simulink model "StraightWithLeadingCar_cs"  (R2016a)
settings: Solver=ode5  SolverMode=SingleTasking  StartTime=0.0  StopTime=40  FixedStep=1/1000  RelTol=1e-3
PreLoadFcn:
  | mbxruntime.callbacks.PreLoadFcn(bdroot);
PostLoadFcn:
  | mbxruntime.callbacks.PostLoadFcn(bdroot);
InitFcn:
  | mbxruntime.callbacks.InitFcn(bdroot);
StartFcn:
  | mbxruntime.callbacks.StartFcn(bdroot);
StopFcn:
  | mbxruntime.callbacks.StopFcn(bdroot);
model workspace (MAT data in the model file):
  mbox_table : struct (value not decoded)
  model_closed = 0
  sim_status = 0
values from neighbouring files (symbols this model uses):
  ACCDuration = 5    [PreScan_Runscript.m]
  V0 = ACCArray(2*ACCCasei-1)    [PreScan_Runscript.m]
  V1 = ACCArray(2*ACCCasei)    [PreScan_Runscript.m]
  VAccuracyIn = 0.8    [PreScan_Runscript.m]
  VDurationIn = 2    [PreScan_Runscript.m]
  VPIDIn = ACCArray(2*ACCCasei-1)    [PreScan_Runscript.m]
  VToleranceIn = 1    [PreScan_Runscript.m]
undefined symbols (not defined in the file or in its folder): ADASID, BMotor1, BMotor2, BrkDelayTime, DControlB, Delay1, Delay2, DiscIntNeverNeededParam, IControlB, JMotor1, JMotor2, mbxruntime, PControlB, PreScanCarSimLoadFcn, ratioGearF, ratioGearR, tabledata, TorqDelayTime, Tstep
undefined symbols (not defined in the file): SteeringColumn, SteeringWheel, WheelL0, WheelL1, WheelR0, WheelR1
libraries: simulink x14, simulink_extras x11, PreScanSimulinkLibrary x9, MyLib x3, Solver_SF x2, PreScanUsefulBlocks x2, pil_lib x1
(part 12 of 12)

== system StraightWithLeadingCar_cs/Roewe_550_S_Sedan_1/CarSim_Vehicle/CarSim2PreScan_BUS/Wheel/Convert CarSim to PreScan Wheel Position/Transformation_WheelGlobal2WheelLocal/PreScan_WheelShiftFR/pos_ini_Visu ==
  Constant : Constant  Value=x_ini_VRML
  Constant1 : Constant  Value=y_ini_VRML
  Constant2 : Constant  Value=TyreRadius-cogZOffset
  Mux1 : Mux  Inputs=3
  pos_ini_Visu : Outport
  wires:
  Constant/1 -> Mux1/1
  Mux1/1 -> pos_ini_Visu/1
  Constant1/1 -> Mux1/2
  Constant2/1 -> Mux1/3

== system StraightWithLeadingCar_cs/Roewe_550_S_Sedan_1/CarSim_Vehicle/CarSim2PreScan_BUS/Wheel/Convert CarSim to PreScan Wheel Position/Transformation_WheelGlobal2WheelLocal/PreScan_WheelShiftRL/pos_ini_Visu ==
  Constant : Constant  Value=-x_ini_VRML
  Constant1 : Constant  Value=y_ini_VRML
  Constant2 : Constant  Value=TyreRadius-cogZOffset
  Mux1 : Mux  Inputs=3
  pos_ini_Visu : Outport
  wires:
  Constant/1 -> Mux1/1
  Mux1/1 -> pos_ini_Visu/1
  Constant1/1 -> Mux1/2
  Constant2/1 -> Mux1/3

== system StraightWithLeadingCar_cs/Roewe_550_S_Sedan_1/CarSim_Vehicle/CarSim2PreScan_BUS/Wheel/Convert CarSim to PreScan Wheel Position/Transformation_WheelGlobal2WheelLocal/PreScan_WheelShiftRR/pos_ini_Visu ==
  Constant : Constant  Value=-x_ini_VRML
  Constant1 : Constant  Value=y_ini_VRML
  Constant2 : Constant  Value=TyreRadius-cogZOffset
  Mux1 : Mux  Inputs=3
  pos_ini_Visu : Outport
  wires:
  Constant/1 -> Mux1/1
  Mux1/1 -> pos_ini_Visu/1
  Constant1/1 -> Mux1/2
  Constant2/1 -> Mux1/3

== system StraightWithLeadingCar_cs/Roewe_550_S_Sedan_1/Subsystem1/CarSim2PreScan_BUS/Wheel/Convert CarSim to PreScan Wheel Position/Transformation_WheelGlobal2WheelLocal/PreScan_WheelShiftFL/pos_ini_Visu ==
  Constant : Constant  Value=x_ini_VRML
  Constant1 : Constant  Value=y_ini_VRML
  Constant2 : Constant  Value=TyreRadius-cogZOffset
  Mux1 : Mux  Inputs=3
  pos_ini_Visu : Outport
  wires:
  Constant2/1 -> Mux1/3
  Constant1/1 -> Mux1/2
  Mux1/1 -> pos_ini_Visu/1
  Constant/1 -> Mux1/1

== system StraightWithLeadingCar_cs/Roewe_550_S_Sedan_1/Subsystem1/CarSim2PreScan_BUS/Wheel/Convert CarSim to PreScan Wheel Position/Transformation_WheelGlobal2WheelLocal/PreScan_WheelShiftFR/pos_ini_Visu ==
  Constant : Constant  Value=x_ini_VRML
  Constant1 : Constant  Value=y_ini_VRML
  Constant2 : Constant  Value=TyreRadius-cogZOffset
  Mux1 : Mux  Inputs=3
  pos_ini_Visu : Outport
  wires:
  Constant/1 -> Mux1/1
  Mux1/1 -> pos_ini_Visu/1
  Constant1/1 -> Mux1/2
  Constant2/1 -> Mux1/3

== system StraightWithLeadingCar_cs/Roewe_550_S_Sedan_1/Subsystem1/CarSim2PreScan_BUS/Wheel/Convert CarSim to PreScan Wheel Position/Transformation_WheelGlobal2WheelLocal/PreScan_WheelShiftRL/pos_ini_Visu ==
  Constant : Constant  Value=-x_ini_VRML
  Constant1 : Constant  Value=y_ini_VRML
  Constant2 : Constant  Value=TyreRadius-cogZOffset
  Mux1 : Mux  Inputs=3
  pos_ini_Visu : Outport
  wires:
  Constant/1 -> Mux1/1
  Mux1/1 -> pos_ini_Visu/1
  Constant1/1 -> Mux1/2
  Constant2/1 -> Mux1/3

== system StraightWithLeadingCar_cs/Roewe_550_S_Sedan_1/Subsystem1/CarSim2PreScan_BUS/Wheel/Convert CarSim to PreScan Wheel Position/Transformation_WheelGlobal2WheelLocal/PreScan_WheelShiftRR/pos_ini_Visu ==
  Constant : Constant  Value=-x_ini_VRML
  Constant1 : Constant  Value=y_ini_VRML
  Constant2 : Constant  Value=TyreRadius-cogZOffset
  Mux1 : Mux  Inputs=3
  pos_ini_Visu : Outport
  wires:
  Constant/1 -> Mux1/1
  Mux1/1 -> pos_ini_Visu/1
  Constant1/1 -> Mux1/2
  Constant2/1 -> Mux1/3

== matlab function StraightWithLeadingCar_cs/Roewe_550_S_Sedan_1/CarSim_Vehicle/CarSim2PreScan_ContactAdapter/Embedded MATLAB Function ==
  data: u input; y output
function y = fcn(u)
%#eml

y = norm(u)/3.6;

== matlab function StraightWithLeadingCar_cs/Roewe_550_S_Sedan_1/CarSim I//O/PreScanLaneMarker/MATLAB Function ==
  data: Lane3_X input; Lane3_Y input; Lane1_X input; Lane1_Y input; Lane2_X input; Lane2_Y input; Lane1 output; Lane2 output; Lane3 output; Lane4_X input; Lane4_Y input; Lane4 output
function [Lane1,Lane2,Lane3,Lane4] = fcn(Lane3_X,Lane3_Y,Lane1_X,Lane1_Y,Lane2_X,Lane2_Y,Lane4_X,Lane4_Y)
%#codegen

p1 = polyfit(Lane1_X,Lane1_Y,3);
p2 = polyfit(Lane2_X,Lane2_Y,3);
p3 = polyfit(Lane3_X,Lane3_Y,3);
p4 = polyfit(Lane4_X,Lane4_Y,3);

Lane1PosC0_m = single(p1(4));
Lane1HeadAngC1_Rad = single(p1(3));
Lane1LaneCurvC2_1pm = single(p1(2));
Lane1CurvDrivC3_1pms = single(p1(1));

Lane2PosC0_m = single(p2(4));
Lane2HeadAngC1_Rad = single(p2(3));
Lane2LaneCurvC2_1pm = single(p2(2));
Lane2CurvDrivC3_1pms = single(p2(1));

Lane3PosC0_m = single(p3(4));
Lane3HeadAngC1_Rad = single(p3(3));
Lane3LaneCurvC2_1pm = single(p3(2));
Lane3CurvDrivC3_1pms = single(p3(1));

Lane4PosC0_m = single(p4(4));
Lane4HeadAngC1_Rad = single(p4(3));
Lane4LaneCurvC2_1pm = single(p4(2));
Lane4CurvDrivC3_1pms = single(p4(1));
% set lane1 and lane3 x to be negtive
Lane1=-1*[Lane1PosC0_m Lane1HeadAngC1_Rad Lane1LaneCurvC2_1pm Lane1CurvDrivC3_1pms];
Lane2=-1*[Lane2PosC0_m Lane2HeadAngC1_Rad Lane2LaneCurvC2_1pm Lane2CurvDrivC3_1pms];
Lane3=-1*[Lane3PosC0_m Lane3HeadAngC1_Rad Lane3LaneCurvC2_1pm Lane3CurvDrivC3_1pms];
Lane4=-1*[Lane4PosC0_m Lane4HeadAngC1_Rad Lane4LaneCurvC2_1pm Lane4CurvDrivC3_1pms];
end

== stateflow chart StraightWithLeadingCar_cs/Roewe_550_S_Sedan_1/CarSim I//O/ACCAEB In/Chart ==
  state Init
    en:
    OnSW=0;
    SetSW=0;
    SpdIncSW=0;
    SpdDecSW=0;
    DisIncSW=0;
    DisDecSW=0;
    CanclSW=0;
    RsmSW=0;
  state CCC
    state CCC_ON
      en:
      OnSW=1;
    state CCC_Set
      en:
      SetSW=1;
    state SpdDec
      en:
      SpdDecSW=1;
      ex:
      SpdDecSW=0;
    state HMIContrl
      en:
      SetSW=0;
    state SpdInc
      en:
      SpdIncSW=1;
      ex:
      SpdIncSW=0;
    state Accomplished
      en:
      OnSW=0;
    (default) -> CCC_ON
    CCC_ON -> CCC_Set : [(SteadyFlag~=0)&&(after(0.5,sec))]
    CCC_Set -> HMIContrl : [after(0.3,sec)]
    HMIContrl -> SpdInc [order 2] : [(SetSpd<V1)&&(after(5,sec))]
    HMIContrl -> SpdDec [order 3] : [(SetSpd>V1)&&(after(5,sec))]
    SpdInc -> HMIContrl : [after(0.3,sec)]
    SpdDec -> HMIContrl : [after(0.3,sec)]
    HMIContrl -> CCC.Accomplished [order 1] : [abs(V0-V1)<5]{after(5,sec)}
  state ACC
    state ACC_ON
      en:
      OnSW=1;
    state ACC_Set
    state SpdBuffer
    state Spd_Dec
    state Spd_Inc
    state Accomplished
    (default) -> ACC_ON
    ACC_ON -> ACC_Set : [SteadyFlag~=0]
    ACC_Set -> SpdBuffer
    SpdBuffer -> Spd_Dec [order 2]
    SpdBuffer -> Spd_Inc [order 1]
    Spd_Dec -> SpdBuffer
    Spd_Inc -> SpdBuffer
    SpdBuffer -> ACC.Accomplished [order 3]
  state LKA
  state TestEnd
  (default) -> Init
  Init -> CCC [order 1] : [ADASID==1]
  Init -> ACC [order 2] : [ADASID==2]
  Init -> LKA [order 3] : [ADASID==3]
  Init -> TestEnd [order 4]
  data: state local; state local; state local; state local; ADASID input; SteadyFlag input; OnSW output; SetSW output; SpdIncSW output; SpdDecSW output; DisIncSW output; DisDecSW output; CanclSW output; RsmSW output; V0 input; V1 input; Interval input; CCCDuration input; HMICounter local; Vtemp local; SetSpd input; MemSpd input

== matlab function StraightWithLeadingCar_cs/Roewe_550_S_Sedan_1/Subsystem1/CarSim2PreScan_ContactAdapter/Embedded MATLAB Function ==
  data: u input; y output
function y = fcn(u)
%#eml

y = norm(u)/3.6;

== stateflow chart StraightWithLeadingCar_cs/Roewe_550_S_Sedan_1/CarSim I//O/ACCAEB In/isSteady/Chart ==
  state NotSteady
    en:
    Counter=0;
    Counter1=0;
  state Steady_ing
    en:
    SteadyFlag=0;
    du:
    Counter = Counter + 1;
  state Steady
    en:
    SteadyFlag=1;
  state SteadyBuffer
    en:
    Counter1=Counter1+1;
    du:
    Counter1=Counter1+1;
  (default) -> NotSteady
  NotSteady -> Steady_ing : [Flag~=0]
  Steady_ing -> Steady [order 2] : [(Counter+Counter1)>VDuration*1000-5]
  SteadyBuffer -> Steady_ing [order 1] : [Flag~=0]
  Steady_ing -> SteadyBuffer [order 1] : [Flag==0]
  SteadyBuffer -> NotSteady [order 2] : [Counter1>VDuration*1000*(1-Accuracy)]
  data: Flag input; SteadyFlag output; Accuracy input; VDuration input; Counter local; Counter1 local

== matlab function StraightWithLeadingCar_cs/Roewe_550_S_Sedan_1/CarSim I//O/Objselect/MATLAB Function2 ==
  data: TIS1_range input; LockX output; TIS1_rangedot input; TIS1_theta input; TIS2_range input; TIS2_rangedot input; TIS2_theta input; PL input; PR input; LockY output; LockVx output; LockID output; flag output
function [LockX,LockY,LockVx,LockID,flag] = fcn(TIS1_range,TIS1_rangedot,TIS1_theta,TIS2_range,TIS2_rangedot,TIS2_theta,PL,PR)
%#codegen

% if T==3.6
%     falg=1;
% end
TIS_range    = [TIS1_range,TIS2_range];
TIS_rangedot = [TIS1_rangedot,TIS2_rangedot];
TIS_theta    = [TIS1_theta,TIS2_theta]*pi()/180;
obj_x        = TIS_range .* cos(TIS_theta);
obj_y        = TIS_range .* sin(TIS_theta);
fitA_y       = polyval(PL,obj_x);
fitB_y       = polyval(PR,obj_x);
flag = 0;
%% make the points to several group

index1      = obj_x>0.01;                               %object in sensor range
index2      = obj_y<=fitA_y & obj_y>=fitB_y & index1;    %object in ego car lane 

if any(index2)~=0;                              %be sure has object in trace
    flag = 1;
    id_xmin           = find(obj_x==min(obj_x(index2)));            %the nearist object in detected
    id_xmin_intrace   = id_xmin(find(index2(id_xmin)==true));       %the nearist object in trace
    LockID            = min(id_xmin_intrace);                       %if more than 2 points get the low ID number
    LockX             = obj_x(LockID);
    LockY             = obj_y(LockID);
    LockVx            = TIS_rangedot(LockID);
else
    LockID            = 0;
    LockX             = 255;
    LockY             = 0;
    LockVx            = 0;
end

== matlab function StraightWithLeadingCar_cs/Roewe_550_S_Sedan_1/CarSim I//O/Objselect/line curve fit1 ==
  data: xl input; pL0 output; yl input; xr input; pL1 output; yr input; pL2 output; pL3 output; pR0 output; pR1 output; pR2 output; pR3 output; pl output; pr output
function [pL0,pL1,pL2,pL3,pR0,pR1,pR2,pR3,pl,pr] = fcn(xl,yl,xr,yr)
%#eml
% pL3 = 0;
% pL2 = 0;
% pL1 = 0;
% pL0 = 0;
% pR3 = 0;
% pR2 = 0;
% pR1 = 0;
% pR0 = 0;

[pl,Sl] = polyfit(xl,yl,3);
pL3 = pl(1);
pL2 = pl(2);
pL1 = pl(3);
pL0 = pl(4);
[pr,Sr] = polyfit(xr,yr,3);
pR3 = pr(1);
pR2 = pr(2);
pR1 = pr(3);
pR0 = pr(4);

if isnan(pL3)
    pL3 = 0;
    pL2 = 0;
    pL1 = 0;
    pL0 = 0;  
end

if isnan(pR3)
    pR3 = 0;
    pR2 = 0;
    pR1 = 0;
    pR0 = 0;  
end
